simulink model "NWMR"  (R2023a)
settings: Solver=VariableStepAuto  StartTime=0.0  StopTime=100  RelTol=1e-3
settings Model: Creator=30296  LastModifiedBy=30296

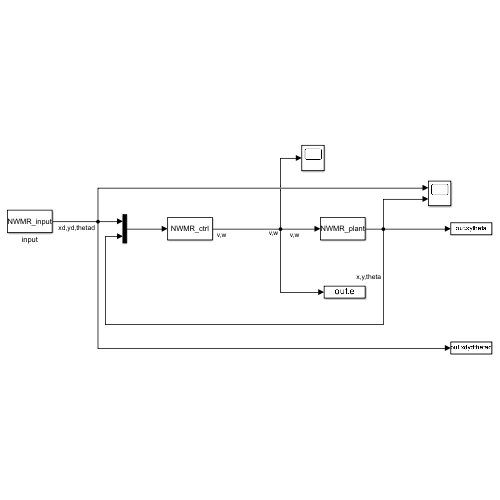
[thumbnail: Simulink's stored preview of the top-level diagram]
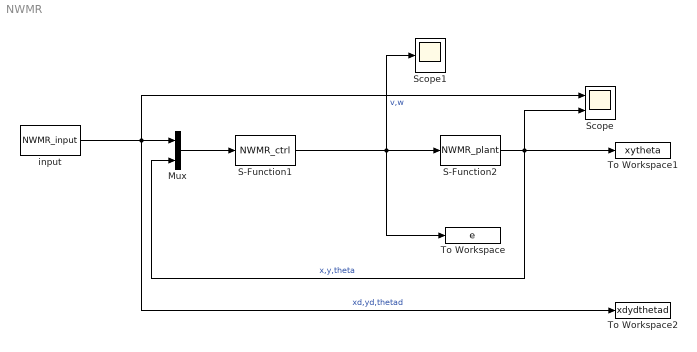
== system NWMR ==
  Mux : Mux  Inputs=2
  S-Function1 : S-Function  FunctionName=NWMR_ctrl  Parameters=pa  SFunctionDeploymentMode=off  EnableBusSupport=off
  S-Function2 : S-Function  FunctionName=NWMR_plant  Parameters=pa  SFunctionDeploymentMode=off  EnableBusSupport=off
  Scope : Scope  NumInputPorts=2
  Scope1 : Scope
  To Workspace : ToWorkspace  VariableName=e  SampleTime=-1
  To Workspace1 : ToWorkspace  VariableName=xytheta  SampleTime=-1
  To Workspace2 : ToWorkspace  VariableName=xdydthetad  SampleTime=-1
  input : S-Function  FunctionName=NWMR_input  Parameters=pa  SFunctionDeploymentMode=off  EnableBusSupport=off
  wires:
  Mux/1 -> S-Function1/1
  input/1 -> To Workspace2/1, Mux/1, Scope/1  "xd,yd,thetad"
  S-Function2/1 -> To Workspace1/1, Mux/2, Scope/2  "x,y,theta"
  S-Function1/1 -> Scope1/1, S-Function2/1, To Workspace/1  "v,w"
